simulink model "MRAC_wing_rock_2_Neel"  (R2019a)
settings: Solver=ode45  StartTime=0.0  StopTime=40  RelTol=1e-3  EnableMultiTasking=on
settings Model: Creator=Administrator  LastModifiedBy=ar-neelabhro.roy
settings DataIOCC: LimitDataPoints=on  SaveFormat=Array  ReturnWorkspaceOutputs=off
settings OptimizationCC: LifeSpan=inf
settings DebuggingCC: SolverPrmCheckMsg=warning  AllowSymbolicDim=off  SFUnexpectedBacktrackingDiag=warning  SFNoUnconditionalDefaultTransitionDiag=warning  SFExecutionAtInitializationDiag=none  ArithmeticOperatorsInVariantConditions=warning
settings HardwareCC: ProdBitPerPointer=32  ProdBitPerSizeT=32  ProdBitPerPtrDiffT=32  ProdLargestAtomicFloat=None  ProdIntDivRoundTo=Undefined  ProdEndianess=Unspecified  ProdWordSize=32  ProdHWDeviceType=32-bit Generic
settings ModelReferenceCC: PropagateSignalLabelsOutOfModel=off
settings SFSimCC: SimUseLocalCustomCode=off
settings RTWCC: RTWUseLocalCustomCode=off
settings CodeAppCC: StateflowObjectComments=on
settings GRTTargetCC: TargetLangStandard=C89/C90 (ANSI)  GeneratePreprocessorConditionals=Disable all
settings ConfigComp: CovMetricSettings=dw  CovHtmlReporting=on  CovSaveCumulativeToWorkspaceVar=on  CovSaveSingleToWorkspaceVar=on  CovExternalEMLEnable=off  CovSFcnEnable=off

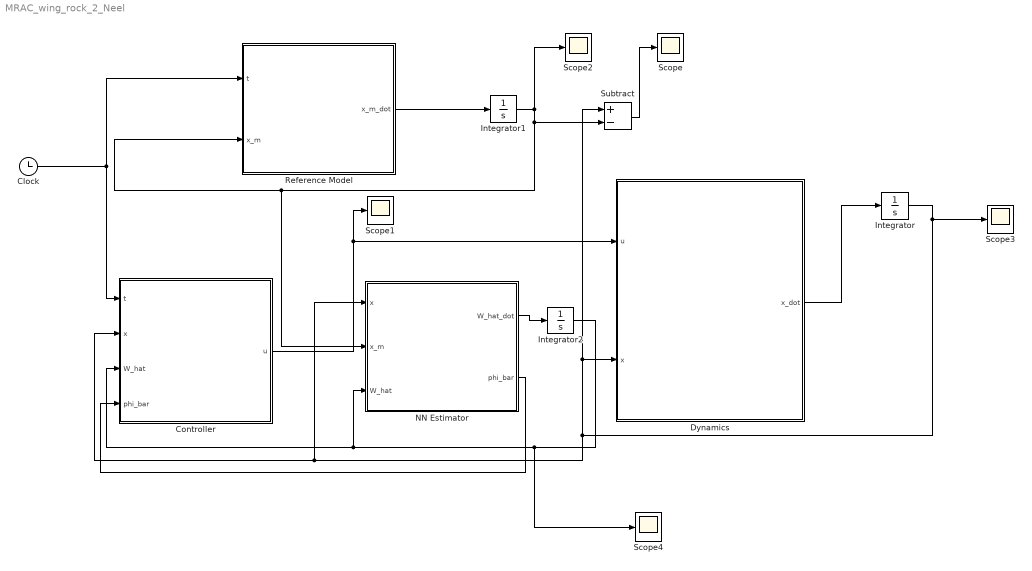
== system MRAC_wing_rock_2_Neel ==
  Clock : Clock
      settings: Decimation=50
  Controller : MATLAB Function  TreatAsAtomicUnit=on
  Dynamics : MATLAB Function  TreatAsAtomicUnit=on
  Integrator : Integrator  InitialCondition=[-1;1]
  Integrator1 : Integrator  InitialCondition=[0;0]
  Integrator2 : Integrator  InitialCondition=zeros(101,1)
  NN Estimator : MATLAB Function  TreatAsAtomicUnit=on
  Reference Model : MATLAB Function  TreatAsAtomicUnit=on
  Scope{,1..4} (5 alike) : Scope
  Subtract : Sum  Inputs=+-
  wires:
  Dynamics/1(x_dot) -> Integrator/1
  Integrator/1 -> Scope3/1, Subtract/1, Dynamics/2(x), NN Estimator/1(x), Controller/2(x)
  Clock/1 -> Controller/1(t), Reference Model/1(t)
  Controller/1(u) -> Scope1/1, Dynamics/1(u)
  Reference Model/1(x_m_dot) -> Integrator1/1
  Integrator1/1 -> Scope2/1, NN Estimator/2(x_m), Reference Model/2(x_m), Subtract/2
  NN Estimator/1(W_hat_dot) -> Integrator2/1
  Integrator2/1 -> Scope4/1, NN Estimator/3(W_hat), Controller/3(W_hat)
  Subtract/1 -> Scope/1
  NN Estimator/2(phi_bar) -> Controller/4(phi_bar)

== matlab function MRAC_wing_rock_2_Neel/Controller ==
  data: u output; t input; x input; W_hat input; phi_bar input
function u  = controller(t,x,W_hat, phi_bar)

%r=10;
%r=exp(-t);
r=sin(t);
%r=2*sin(t);

k_x=[-2/3 -1/3]'; % note that the linear control gain is directly chosen instead of adapting with an assumption of $A$ matrix to be known


u=k_x'*x+r-W_hat'*phi_bar;

end

== matlab function MRAC_wing_rock_2_Neel/Dynamics ==
  data: u input; x input; x_dot output
function x_dot   = dynamics(u,x)
%#codegen
L_delta_a=3;
A=[0 1; 0 0];
B=[0;L_delta_a];
a0=0.8;
a1=0.2314;
a2=0.6918;
a3=-0.6245;
a4=0.0095;
a5=0.0214;

theta=x(1,1);
p=x(2,1);

delta=a0+a1*theta+a2*p+a3*abs(theta)*p+a4*abs(p)*p+a5*theta^3;
x_dot=A*x+B*(u+delta/L_delta_a);
end

== matlab function MRAC_wing_rock_2_Neel/NN Estimator ==
  data: W_hat_dot output; x input; x_m input; phi_bar output; W_hat input
function [W_hat_dot, phi_bar]   = NN_estimator(x,x_m,W_hat)

e=x-x_m; % tracking error 
sigma = 2;


L=100; % number of neurons
Gamma=1*eye(L+1);
phi=zeros(L,1);
Vr=5*eye(size(x,1)); % variance of RBF

%For L=5
%C=[0.6294   -0.7460    0.2647   -0.4430    0.9150;
%    0.8116    0.8268   -0.8049    0.0938    0.9298];

%For L=10
%C=[-0.6848    0.9143    0.6006   -0.1565    0.5844    0.3115    0.6983    0.3575    0.4863    0.3110
%    0.9412   -0.0292   -0.7162    0.8315    0.9190   -0.9286    0.8680    0.5155   -0.2155   -0.6576]; %L=10

%For L=100
C = [0.629447372786358,-0.746026367412988,0.264718492450819,-0.443003562265903,0.915013670868595,-0.684773836644903,0.914333896485891,0.600560937777600,-0.156477434747450,0.584414659119109,0.311481398313174,0.698258611737554,0.357470309715547,0.486264936249832,0.310955780355113,0.412092176039218,-0.446154030078220,-0.805736437528305,0.389657245951634,0.900444097676710,-0.122511280687204,0.531033576298005,-0.626254790891243,-0.108827598578201,0.418729661716145,-0.447949846002843,0.310196007947681,-0.762004636883247,0.919487917032162,0.170535501959555,0.502534118611306,0.0119141033302848,0.781806505071597,0.0944310599276061,-0.701411988881885,0.681434511967325,0.628569652137633,0.858527246374456,-0.606809499137584,0.232089352293278,-0.296680985874007,0.170528182305449,0.834387327659620,0.514400458221443,-0.239108306049287,-0.848291420873873,0.0615951060179454,0.868021368458366,0.137647321744385,-0.976195860997517,-0.675635383613515,-0.377569915910390,-0.668702541000438,-0.474057430919711,0.378429006280016,-0.0989168029950045,-0.542046062566362,-0.695243962061554,0.0766848705201142,-0.843648942493633,-0.786694459638831,-0.990731551731865,0.634606441306866,-0.831128308978179,-0.480259194298692,-0.137172345072911,-0.636305943394295,-0.708922039230566,0.738584415280179,0.0997204036726640,0.706062235443787,-0.298095238215458,-0.196383932496117,-0.520167692892684,-0.632184423435167,-0.165465861831261,0.805432219830562,-0.0182718150638401,-0.324561180357246,-0.261506437759570,0.560504136642276,-0.516617428172335,-0.807090949663223,0.884101181550970,0.150417190156931,-0.530440173255187,0.642388080395918,-0.913952396684384,0.298230949912904,0.295491926272613,0.0940177845726899,0.489385614148312,0.373550866730630,-0.263030807019327,0.560454870302754,0.858771941937460,-0.0264167351936553,-0.106432501140387,0.0170173107622540,0.635255416644524
    0.811583874151238,0.826751712278039,-0.804919190001181,0.0937630384099677,0.929777070398553,0.941185563521231,-0.0292487025543176,-0.716227322745569,0.831471050378134,0.918984852785806,-0.928576642851621,0.867986495515101,0.515480261156667,-0.215545960931664,-0.657626624376877,-0.936334307245159,-0.907657218737692,0.646915656654585,-0.365801039878279,-0.931107838994183,-0.236883085813983,0.590399802274126,-0.0204712084235379,0.292626020222529,0.509373363964722,0.359405353707350,-0.674776529610739,-0.00327189603571409,-0.319228546667734,-0.552376121017726,-0.489809769081462,0.398153445313372,0.918582850410889,-0.722751114342642,-0.484983491752527,-0.491435642056938,-0.512950062550021,-0.300032468030383,-0.497832284047938,-0.0534223021945415,0.661657255792582,0.0994472165822791,-0.428321962359253,0.507458188556991,0.135643281450442,-0.892099762666786,0.558334460204022,-0.740187583052540,-0.0612187178835884,-0.325754711202237,0.588569081367814,0.0570662710124255,0.203963882803273,0.308158196953565,0.496303185647419,-0.832357244006135,0.826674723003339,0.651633954979095,0.992269433253771,-0.114643460449107,0.923796161710107,0.549820929423005,0.737389410727019,-0.200434701802207,0.600136960448615,0.821295188859046,-0.472394166956020,-0.727862882582673,0.159409174731140,-0.710090403552546,0.244110262970132,0.0264990797341067,-0.848066616618316,-0.753362130329669,-0.520094948670195,-0.900691139348516,0.889574379443292,-0.0214947231999623,0.800107692835324,-0.777594489412425,-0.220522326077493,-0.192175708823771,-0.736053414787330,0.912269080459605,-0.880440914105688,-0.293682857555858,-0.969193124696890,-0.662019941074591,0.463444771317341,-0.0981525871381102,-0.407358388784454,-0.622089969934911,-0.632977688525461,0.251237121459381,-0.837748462268430,0.551425357216805,-0.128282822838162,-0.387301055966885,0.0215431283442193,0.589662833766906]; %L = 100



for i=1:L
    phi(i,1)=exp(-((x-C(:,i))'*(Vr\(x-C(:,i)))));
end
phi_bar=[1;phi];


P=[3.5 0.5; 0.5 1.5]; % the command P=lyap(A_m',Q) is used to calculate P. In this case Q is chosen as Q=2*eye(2). 
L_delta_a=3;
B=[0;L_delta_a];


%W_hat_dot=Gamma*phi_bar*e'*P*B;                                %Without Robust Modification
%W_hat_dot=Gamma*(phi_bar*e'*P*B -sigma*W_hat);                %For Sigma Modification
W_hat_dot=Gamma*(phi_bar*e'*P*B -sigma*(norm(e'*P*B))*W_hat); %For e Modification

== matlab function MRAC_wing_rock_2_Neel/Reference Model ==
  data: x_m_dot output; t input; x_m input
function x_m_dot  = reference(t,x_m)
am1=-2;
am2=-1;
L_delta_a=3;
%r=exp(-t);
r=sin(t);
%r=2*sin(t);
A_m=[0 1; am1 am2];
B_m=[0; L_delta_a];
x_m_dot=A_m*x_m+B_m*r;
